simulink library "uav_utilities"  (Simulink 7.1)
values from neighbouring files (symbols this model uses):
  I = find(Ev == Ev(1))    [res_power_junction_m.m]
undefined symbols (not defined in the file or in its folder): euler_0, g, inner_sysd, K_inner, K_outer, Kx_inner, KX_outer, Ky_inner, KY_outer, L, m, omega_0, outer_sysd, pow_gps_pos_sim, pow_gps_vel_sim, pow_imu_pos_sim, pow_imu_rate_sim, pow_sodar_sim, t_comp_inner, t_comp_outer, t_gps, t_imu, t_inner, t_outer, t_sodar, tau, thrust_max, torque_max, Vb_0, XYZ_0
libraries: simulink x33, aero_sim_lib x9, aerolibprivatev1p5 x1
(part 3 of 3)

== system uav_utilities/STARMAC/gum_stix/sensor_fusion/if_end/If Action Subsystem1 ==
  Xe_sh_1p : Inport  OutDataType=sfix(16)  OutScaling=2^0
  dX_1p : Inport  Port=2  OutDataType=sfix(16)  OutScaling=2^0
  Action Port : ActionPort  InitializeStates=reset
  Xe_sh_1 : Outport  DataType=single  OutDataType=sfix(16)  OutScaling=2^0  OutDataTypeStr=single  OutputWhenDisabled=reset  InitialOutput=zeros(1,3,'single')
  dX_1 : Outport  Port=2  DataType=single  OutDataType=sfix(16)  OutScaling=2^0  OutDataTypeStr=single  OutputWhenDisabled=reset  InitialOutput=zeros(1,3,'single')
  wires:
  Xe_sh_1p/1 -> Xe_sh_1/1
  dX_1p/1 -> dX_1/1

== system uav_utilities/STARMAC/gum_stix/sensor_fusion/if_end1/If Action Subsystem ==
  Ve_s : Inport  OutDataType=sfix(16)  OutScaling=2^0
  Ve_f : Inport  Port=2  OutDataType=sfix(16)  OutScaling=2^0
  Action Port : ActionPort  InitializeStates=reset
  Sum : Sum  Inputs=-+|  OutDataTypeMode=single  OutDataType=sfix(16)  OutScaling=2^0  OutDataTypeStr=single
  Ve_sh_1 : Outport  OutDataType=sfix(16)  OutScaling=2^0  OutputWhenDisabled=reset  InitialOutput=zeros(1,3,'single')
  dV_1 : Outport  Port=2  OutDataType=sfix(16)  OutScaling=2^0  OutputWhenDisabled=reset  InitialOutput=zeros(1,3,'single')
  wires:
  Ve_s/1 -> Ve_sh_1/1, Sum/1
  Ve_f/1 -> Sum/2
  Sum/1 -> dV_1/1

== system uav_utilities/STARMAC/gum_stix/sensor_fusion/if_end1/If Action Subsystem1 ==
  Ve_sh_1p : Inport  OutDataType=sfix(16)  OutScaling=2^0
  dV_1p : Inport  Port=2  OutDataType=sfix(16)  OutScaling=2^0
  Action Port : ActionPort  InitializeStates=reset
  Ve_sh_1 : Outport  DataType=single  OutDataType=sfix(16)  OutScaling=2^0  OutDataTypeStr=single  OutputWhenDisabled=reset  InitialOutput=zeros(1,3,'single')
  dV_1 : Outport  Port=2  DataType=single  OutDataType=sfix(16)  OutScaling=2^0  OutDataTypeStr=single  OutputWhenDisabled=reset  InitialOutput=zeros(1,3,'single')
  wires:
  dV_1p/1 -> dV_1/1
  Ve_sh_1p/1 -> Ve_sh_1/1

== system uav_utilities/STARMAC/starmac_dynamics/starmac_blade_flapping_effects/starmac_body_moments/CrossProduct(AXB) ==
  A : Inport  OutDataType=sfix(16)  OutScaling=2^0
  B : Inport  Port=2  OutDataType=sfix(16)  OutScaling=2^0
  Fcn : Fcn  Expr=u[2]*u[6]-u[3]*u[5]
  Fcn1 : Fcn  Expr=u[3]*u[4]-u[1]*u[6]
  Fcn2 : Fcn  Expr=u[1]*u[5]-u[2]*u[4]
  Mux : Mux  Inputs=2
  Mux1 : Mux  Inputs=3
  Out : Outport  OutDataType=sfix(16)  OutScaling=2^0
  wires:
  A/1 -> Mux/1
  B/1 -> Mux/2
  Mux/1 -> Fcn/1, Fcn1/1, Fcn2/1
  Fcn/1 -> Mux1/1
  Fcn1/1 -> Mux1/2
  Fcn2/1 -> Mux1/3
  Mux1/1 -> Out/1

== system uav_utilities/STARMAC/starmac_dynamics/starmac_blade_flapping_effects/starmac_body_moments/CrossProduct(AXB)1 ==
  A : Inport  OutDataType=sfix(16)  OutScaling=2^0
  B : Inport  Port=2  OutDataType=sfix(16)  OutScaling=2^0
  Fcn : Fcn  Expr=u[2]*u[6]-u[3]*u[5]
  Fcn1 : Fcn  Expr=u[3]*u[4]-u[1]*u[6]
  Fcn2 : Fcn  Expr=u[1]*u[5]-u[2]*u[4]
  Mux : Mux  Inputs=2
  Mux1 : Mux  Inputs=3
  Out : Outport  OutDataType=sfix(16)  OutScaling=2^0
  wires:
  Mux1/1 -> Out/1
  Fcn2/1 -> Mux1/3
  Fcn1/1 -> Mux1/2
  Fcn/1 -> Mux1/1
  Mux/1 -> Fcn2/1, Fcn1/1, Fcn/1
  B/1 -> Mux/2
  A/1 -> Mux/1

== system uav_utilities/STARMAC/starmac_dynamics/starmac_blade_flapping_effects/starmac_body_moments/CrossProduct(AXB)2 ==
  A : Inport  OutDataType=sfix(16)  OutScaling=2^0
  B : Inport  Port=2  OutDataType=sfix(16)  OutScaling=2^0
  Fcn : Fcn  Expr=u[2]*u[6]-u[3]*u[5]
  Fcn1 : Fcn  Expr=u[3]*u[4]-u[1]*u[6]
  Fcn2 : Fcn  Expr=u[1]*u[5]-u[2]*u[4]
  Mux : Mux  Inputs=2
  Mux1 : Mux  Inputs=3
  Out : Outport  OutDataType=sfix(16)  OutScaling=2^0
  wires:
  A/1 -> Mux/1
  B/1 -> Mux/2
  Mux/1 -> Fcn/1, Fcn1/1, Fcn2/1
  Fcn/1 -> Mux1/1
  Fcn1/1 -> Mux1/2
  Fcn2/1 -> Mux1/3
  Mux1/1 -> Out/1

== system uav_utilities/STARMAC/starmac_dynamics/starmac_blade_flapping_effects/starmac_body_moments/CrossProduct(AXB)3 ==
  A : Inport  OutDataType=sfix(16)  OutScaling=2^0
  B : Inport  Port=2  OutDataType=sfix(16)  OutScaling=2^0
  Fcn : Fcn  Expr=u[2]*u[6]-u[3]*u[5]
  Fcn1 : Fcn  Expr=u[3]*u[4]-u[1]*u[6]
  Fcn2 : Fcn  Expr=u[1]*u[5]-u[2]*u[4]
  Mux : Mux  Inputs=2
  Mux1 : Mux  Inputs=3
  Out : Outport  OutDataType=sfix(16)  OutScaling=2^0
  wires:
  Mux1/1 -> Out/1
  Fcn2/1 -> Mux1/3
  Fcn1/1 -> Mux1/2
  Fcn/1 -> Mux1/1
  Mux/1 -> Fcn2/1, Fcn1/1, Fcn/1
  B/1 -> Mux/2
  A/1 -> Mux/1

== system uav_utilities/STARMAC/starmac_dynamics/starmac_blade_flapping_effects/starmac_body_moments/Motor Thrust to Torques ==
  Thrusts : Inport  OutDataType=sfix(16)  OutScaling=2^0
  Demux : Demux
  Gain1 : Gain  Gain=K_torque  ParameterDataType=sfix(16)  ParameterScaling=2^0  OutDataType=sfix(16)  OutScaling=2^0
  torque 1 : Outport  OutDataType=sfix(16)  OutScaling=2^0
  torque 2 : Outport  Port=2  OutDataType=sfix(16)  OutScaling=2^0
  torque 3 : Outport  Port=3  OutDataType=sfix(16)  OutScaling=2^0
  torque 4 : Outport  Port=4  OutDataType=sfix(16)  OutScaling=2^0
  wires:
  Thrusts/1 -> Gain1/1
  Gain1/1 -> Demux/1
  Demux/1 -> torque 1/1
  Demux/2 -> torque 2/1
  Demux/3 -> torque 3/1
  Demux/4 -> torque 4/1

== matlab function STARMAC/gum_stix/body_to_inertial/Ab_to_Ae ==
  data: euler input single size=[3]; Ae output single size=[3]; Ab input single size=[3]
function Ae = fcn(euler, Ab)
% This block supports the Embedded MATLAB subset.
% See the help menu for details. 
phi=euler(1);
theta=euler(2);
psi=euler(3);
c_phi=cos(phi);
c_theta=cos(theta);
c_psi=cos(psi);
s_phi=sin(phi);
s_theta=sin(theta);
s_psi=sin(psi);
R=single([c_theta*c_psi, c_theta*s_psi, -s_theta;
   s_phi*s_theta*c_psi-c_phi*s_psi, s_phi*s_theta*s_psi+c_phi*c_psi, c_theta*s_phi;
   c_phi*s_theta*c_psi+s_phi*s_psi, c_phi*s_theta*s_psi-s_phi*c_psi, c_theta*c_phi]);
%R=single(zeros(3,3));
%R(1,1)=c_theta*c_psi;
%R(1,2)=c_theta*s_psi;
%R(1,3)=-s_theta;
%R(2,1)=s_phi*s_theta*c_psi - c_phi*s_psi;
%R(2,2)=s_phi*s_theta*s_psi + c_phi*c_psi;
%R(2,3)=c_theta*s_phi;
%R(3,1)=c_phi*s_theta*c_psi + s_phi*s_psi;
%R(3,2)=c_phi*s_theta*s_psi - s_phi*c_psi;
%R(3,3)=c_theta*c_phi;
Ae= transpose(R) * Ab;
%Ae= single(Aed);

== matlab function STARMAC/gum_stix/inertial_pos_controller/demux_fc_xyz ==
  data: fc_xyz input single size=[3]; fc_x output single size=[1]; fc_y output single size=[1]; fc_z output single size=[1]
function [fc_x,fc_y, fc_z] = fcn(fc_xyz)
% This block supports the Embedded MATLAB subset.
% See the help menu for details. 
fc_x=fc_xyz(1);
fc_y=fc_xyz(2);
fc_z=fc_xyz(3);

== matlab function STARMAC/gum_stix/inertial_pos_controller/mux_euler ==
  data: ficx_ficz input single size=[1]; euler output single size=[3]; ficy_ficz input single size=[1]; psi_a input single size=[1]; psi_s input single
function euler = fcn(ficx_ficz, ficy_ficz, psi_a, psi_s)
% This block supports the Embedded MATLAB subset.
% See the help menu for details. 

A = [sin(psi_a) -cos(psi_a); cos(psi_a) sin(psi_a)];
% Get [phi, theta] 
euler_angs = (A * [ficx_ficz; ficy_ficz])';

euler=[euler_angs(1);euler_angs(2);psi_s];

== matlab function STARMAC/gum_stix/rate_limiter/Embedded MATLAB Function ==
  data: Xd input single; Xr output single; Xd_prev input single; Tsamp input single; Vmax input single
function Xr = limit_rate(Xd, Xd_prev, Tsamp, Vmax)
% This block supports the Embedded MATLAB subset.
% See the help menu for details. 

delta = Xd - Xd_prev;
delta = sign(delta) .* min( abs(delta), (ones(size(delta)) * Tsamp * Vmax) );

Xr = Xd_prev + delta;

== matlab function STARMAC/robo_stix/u_T_u_torque_motor_thrust/u_torque_u_T_mux ==
  data: u_torque input single size=[3]; u_torque_u_T output single size=[4]; u_T input single size=[1]
function u_torque_u_T = fcn(u_torque, u_T)
% This block supports the Embedded MATLAB subset.
% See the help menu for details. 
u_torque_u_T = [u_torque; u_T];
